simulink model "exnb4137986_Q7"  (R2023b)
settings: Solver=FixedStepAuto  StartTime=0  StopTime=100  FixedStep=0.01  RelTol=1e-3
values from neighbouring files (symbols this model uses):
  B = double([diff(Xdot(1), u) ... (first row only)    [exnb4137986_Q10.m]    (also in exnb4137986_Q7.m; exnb4137986_Q8.m; exnb4137986_Q9.m)
  xeq2 = double([eq.x1(2) ... (first row only)    [exnb4137986_Q10.m]    (also in exnb4137986_Q7.m; exnb4137986_Q8.m; exnb4137986_Q9.m)
settings Model: Creator=therk  LastModifiedBy=therk

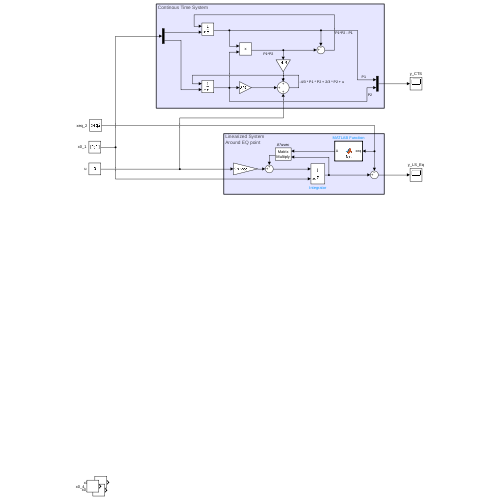
[thumbnail: Simulink's stored preview of the top-level diagram]
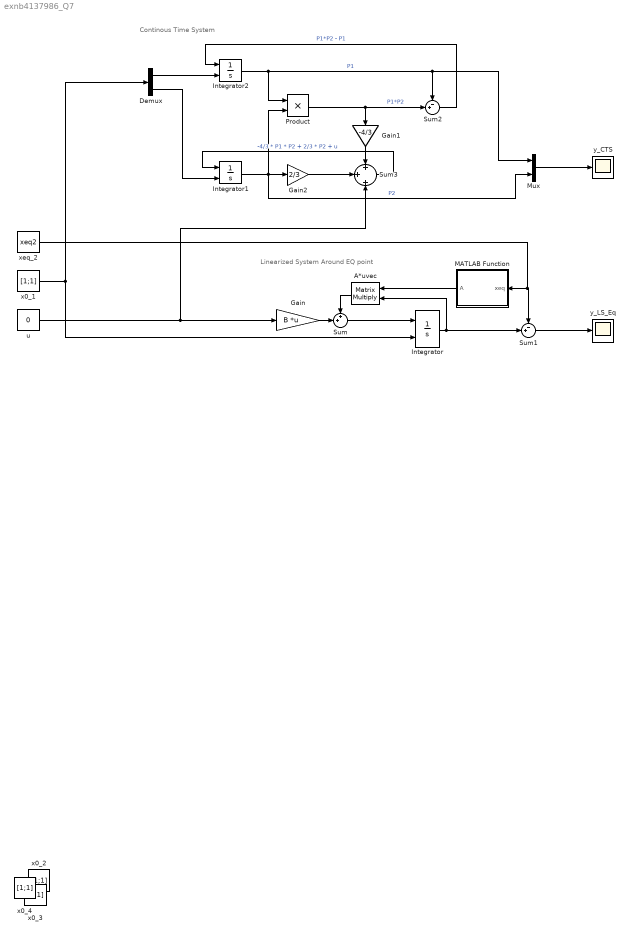
== system exnb4137986_Q7 ==
  note: Continous Time System
  note: Linearized System
      | Around EQ point
  A*uvec : Product  Multiplication=Matrix(*)
  Demux : Demux  Outputs=2
  Gain : Gain  Gain=B  Multiplication=Matrix(K*u) (u vector)
  Gain1 : Gain  Gain=-4/3
  Gain2 : Gain  Gain=2/3
  Integrator : Integrator  InitialConditionSource=external  InitialCondition=[0.5;0]
  Integrator1 : Integrator  InitialConditionSource=external
  Integrator2 : Integrator  InitialConditionSource=external
  MATLAB Function : MATLAB Function  TreatAsAtomicUnit=on
  Mux : Mux  Inputs=2
  Product : Product
  Sum : Sum  Inputs=++|
  Sum1 : Sum  Inputs=-+|
  Sum2 : Sum  Inputs=-+|
  Sum3 : Sum  Inputs=+|+|+
  u : Constant  Value=0
  x0_{1..4} (4 alike) : Constant  Value=[1;1]
  xeq_2 : Constant  Value=xeq2
  y_CTS : Scope
  y_LS_Eq : Scope
  wires:
  Sum1/1 -> y_LS_Eq/1
  xeq_2/1 -> MATLAB Function/1(xeq), Sum1/1
  A*uvec/1 -> Sum/1
  MATLAB Function/1(A) -> A*uvec/1
  Sum/1 -> Integrator/1
  Gain/1 -> Sum/2
  Integrator/1 -> Sum1/2, A*uvec/2
  Mux/1 -> y_CTS/1
  Demux/1 -> Integrator2/2
  Demux/2 -> Integrator1/2
  Integrator1/1 -> Gain2/1, Mux/2, Product/2  "P2"
  Integrator2/1 -> Mux/1, Sum2/1, Product/1  "P1"
  x0_1/1 -> Integrator/2, Demux/1
  Product/1 -> Sum2/2, Gain1/1  "P1*P2"
  Sum3/1 -> Integrator1/1  "-4/3 * P1 * P2 + 2/3 * P2 + u"
  Sum2/1 -> Integrator2/1  "P1*P2 - P1"
  u/1 -> Sum3/3, Gain/1
  Gain2/1 -> Sum3/2
  Gain1/1 -> Sum3/1

== matlab function exnb4137986_Q7/MATLAB Function ==
  data: A output; xeq input
function A = fcn(xeq)
    A = computeA(xeq(1), xeq(2));
end
